simulink model "sampleModel1591"  (R2023a)
settings: Solver=VariableStepAuto  StartTime=0.0  StopTime=10.0  RelTol=1e-3
libraries: hdlsllib x7, simulink x2
settings Model: Creator=user1  LastModifiedBy=user1

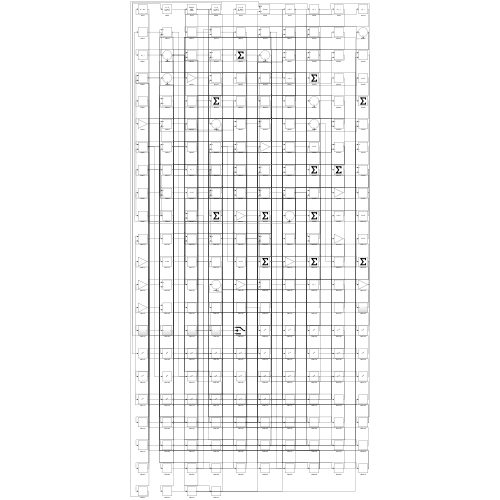
[thumbnail: Simulink's stored preview of the top-level diagram]
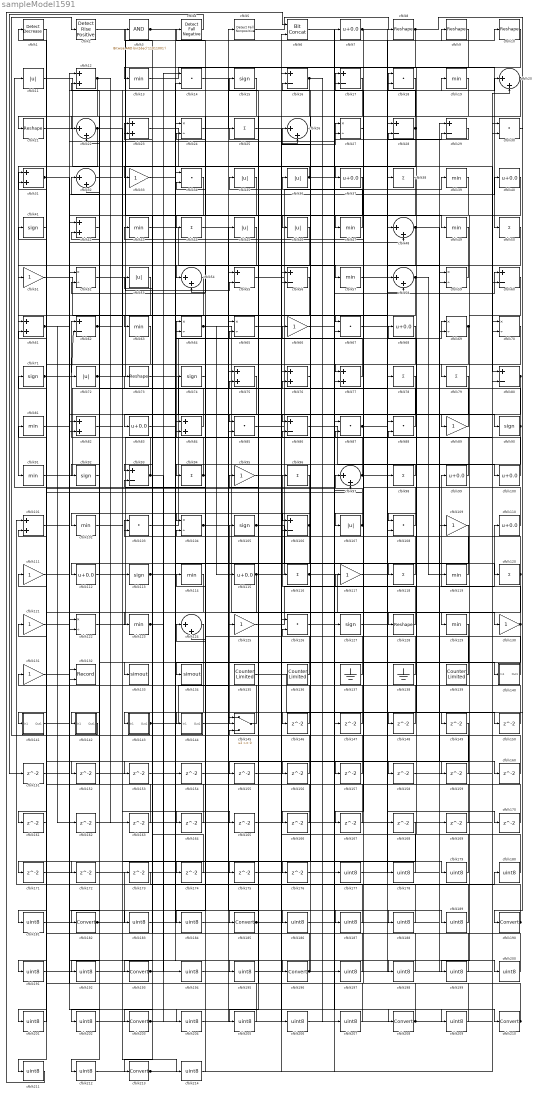
== system sampleModel1591 ==
  cfblk1 : simulink/Logic and Bit Operations/Detect Decrease  vinit=0.0  OutDataTypeStr=boolean
      settings: LibrarySourceBlock=|
      | hdlsllib/Logic and Bit
      | Operations/Detect
      | Decrease
  cfblk{8..10,21,73,128} (6 alike) : Reshape
  cfblk{7,37,40,68,83,99..100,110,112,115} (10 alike) : Bias  Bias=0.0  SaturateOnIntegerOverflow=off
  cfblk{12,23,31,42,61,75..77,82,84,101} (11 alike) : Sum
  cfblk{13,19,39,43,47,49,57,63,81,91,102,114,119,123,129} (15 alike) : MinMax
  cfblk{14,18,30,34,67,85,87..88,103,108,126} (11 alike) : DotProduct  OutDataTypeStr=Inherit: Inherit via internal rule
  cfblk{24,27,52,59,64..65,69..70,104,122} (10 alike) : Product  Inputs=*/  RndMeth=Zero  SaturateOnIntegerOverflow=on
  cfblk{15,41,71,74,90,92,105,113,127} (9 alike) : Signum
  cfblk{16..17,28..29,55..56,60,62,80,86,93,106} (12 alike) : Sum  Inputs=+-
  cfblk{11,35..36,45..46,53,72,107} (8 alike) : Abs  SaturateOnIntegerOverflow=off
  cfblk{33,51,66,89,95,109,111,117,121,125,130..131} (12 alike) : Gain
  cfblk{25,38,44,50,78..79,94,96,98,116,118,120} (12 alike) : Sum  Inputs=+
  cfblk{20,22,26,32,48,54,58,97,124} (9 alike) : Sum  Inputs=|++
  cfblk132 : Record  FileSettingsInternal="{\"entries\":[{\"content\":{\"excelSettings\":{\"content\":{},\"type\":\"Streamout.ExcelSettings\"}},\"type\":\"Streamout.FileSettingStorage\",\"uuid\":\"\"}],\"packageUris\":[\"http:\\/\\/schema.mathworks.com\\/mf0\\/streamout_blocks\\/R2020a\"],\"version\":\"1.0\"}"  Layout=[1 1]  SignalsInternal="{\"entries\":[{\"content\":{\"signals\":[{\"content\":{\"blockPath\":[],\"dimensions\":[1],\"domain\":\"\",\"lineColor\":\"#a2142f\",\"plots\":[1],\"port\":1,\"signalID\":2166,\"signalName\":\"XY Graph:1\"},\"type\":\"RecordBlkView.Signal\",\"uuid\":\"\"},{\"content\":{\"blockPath\":[],\"dimensions\":[1],\"domain\":\"\",\"lineColor\":\"#139fff\",\"plots\":[1],\"port\":2,\"signalID\":2169,\"signalName\":\"XY Graph:2\"},\"type\":\"RecordBlkView.Signal\",\"uuid\":\"\"}]},\"type\":\"RecordBlkView.InputSignals\",\"uuid\":\"\"}],\"packageUris\":[\"http:\\/\\/schema.mathworks.com\\/mf0\\/streamout_blocks\\/R2020a\"],\"version\":\"1.0\"}"  VisualizationBindings="{\"xyplotplugin\":{\"info\":[{\"series\":[{\"bindingParametersList\":[{\"parameter\":\"X-Axis\",\"signalID\":2166,\"signalName\":\"XY Graph:1\"},{\"parameter\":\"Y-Axis\",\"signalID\":2169,\"signalName\":\"XY Graph:2\"}],\"seriesID\":32629}],\"subplotID\":1}]}}"  CompatibilityTag=XY  st=-1
  cfblk133 : ToWorkspace  VariableName=simout  SaveFormat=Timeseries  SampleTime=-1
  cfblk134 : ToWorkspace  VariableName=simout  SaveFormat=Timeseries  SampleTime=-1
  cfblk135 : hdlsllib/Sources/Counter Limited  uplimit=7  tsamp=-1
  cfblk136 : hdlsllib/Sources/Counter Limited  uplimit=7  tsamp=-1
  cfblk137 : Ground
  cfblk138 : Ground
  cfblk139 : hdlsllib/Sources/Counter Limited  uplimit=7  tsamp=-1
  cfblk140 : Subsystem
      settings: LibrarySourceBlock=|
      | hdlsllib/Ports &
      | Subsystems/Subsystem
  cfblk141 : Subsystem
      settings: LibrarySourceBlock=|
      | hdlsllib/Ports &
      | Subsystems/Subsystem
  cfblk142 : Subsystem
      settings: LibrarySourceBlock=|
      | hdlsllib/Ports &
      | Subsystems/Subsystem
  cfblk143 : Subsystem
      settings: LibrarySourceBlock=|
      | hdlsllib/Ports &
      | Subsystems/Subsystem
  cfblk144 : Subsystem
      settings: LibrarySourceBlock=|
      | hdlsllib/Ports &
      | Subsystems/Subsystem
  cfblk145 : Switch  SaturateOnIntegerOverflow=off  InputSameDT=off
  cfblk{146..176} (31 alike) : Delay  SampleTime=1
  cfblk{177..181,183..184,186..189,191..192,194..195,197..202,204..207,209,211..212,214} (29 alike) : DataTypeConversion  OutDataTypeStr=uint8  SaturateOnIntegerOverflow=off  RndMeth=Floor
  cfblk{182,185,190,193,196,203,208,210,213} (9 alike) : DataTypeConversion  SaturateOnIntegerOverflow=off  RndMeth=Floor
  cfblk2 : hdlsllib/Logic and Bit Operations/Detect Rise Positive  vinit=0  OutDataTypeStr=boolean
  cfblk3 : simulink/Logic and Bit Operations/Bitwise Operator  logicop=AND  UseBitMask=on  BitMask=bin2dec('11011001')  BitMaskRealWorld=Stored Integer
      settings: LibrarySourceBlock=|
      | hdlsllib/Logic and Bit
      | Operations/Bitwise
      | Operator
  cfblk4 : hdlsllib/Logic and Bit Operations/Detect Fall Negative  vinit=0  OutDataTypeStr=boolean
  cfblk5 : hdlsllib/Logic and Bit Operations/Detect Fall Nonpositive  vinit=0  OutDataTypeStr=boolean
  cfblk6 : hdlsllib/Logic and Bit Operations/Bit Concat  numInputs=2
  wires:
  cfblk22/1 -> cfblk91/1, cfblk85/1, cfblk165/1, cfblk200/1
  cfblk100/1 -> cfblk62/1
  cfblk105/1 -> cfblk118/1, cfblk27/2
  cfblk115/1 -> cfblk39/1, cfblk123/1
  cfblk72/1 -> cfblk9/1, cfblk20/1
  cfblk13/1 -> cfblk50/1
  cfblk5/1 -> cfblk8/1
  cfblk137/1 -> cfblk11/1
  cfblk125/1 -> cfblk110/1
  cfblk73/1 -> cfblk90/1
  cfblk75/1 -> cfblk193/1
  cfblk108/1 -> cfblk43/1
  cfblk114/1 -> cfblk213/1
  cfblk42/1 -> cfblk112/1
  cfblk1/1 -> cfblk21/1
  cfblk122/1 -> cfblk97/1
  cfblk71/1 -> cfblk62/2, cfblk183/1
  cfblk64/1 -> cfblk130/1, cfblk115/1
  cfblk53/1 -> cfblk141/1(In1)
  cfblk116/1 -> cfblk129/1, cfblk60/1
  cfblk8/1 -> cfblk143/1(In1), cfblk13/1
  cfblk78/1 -> cfblk107/1
  cfblk107/1 -> cfblk31/1, cfblk71/1
  cfblk89/1 -> cfblk64/1
  cfblk113/1 -> cfblk69/1, cfblk195/1
  cfblk103/1 -> cfblk29/1
  cfblk92/1 -> cfblk142/1(In1)
  cfblk59/1 -> cfblk54/1
  cfblk99/1 -> cfblk74/1
  cfblk128/1 -> cfblk96/1
  cfblk16/1 -> cfblk44/1, cfblk205/1, cfblk207/1
  cfblk140/1(Out1) -> cfblk68/1
  cfblk145/1 -> cfblk81/1
  cfblk2/1 -> cfblk49/1
  cfblk90/1 -> cfblk16/2, cfblk148/1
  cfblk76/1 -> cfblk106/1
  cfblk12/1 -> cfblk61/1, cfblk163/1
  cfblk131/1 -> cfblk196/1
  cfblk69/1 -> cfblk77/1, cfblk122/2
  cfblk34/1 -> cfblk63/1
  cfblk48/1 -> cfblk133/1, cfblk132/2, cfblk160/1
  cfblk51/1 -> cfblk98/1
  cfblk83/1 -> cfblk84/1
  cfblk142/1(Out1) -> cfblk2/1
  cfblk47/1 -> cfblk15/1
  cfblk93/1 -> cfblk72/1, cfblk194/1
  cfblk14/1 -> cfblk89/1
  cfblk118/1 -> cfblk64/2
  cfblk21/1 -> cfblk80/1
  cfblk87/1 -> cfblk149/1, cfblk150/1
  cfblk38/1 -> cfblk46/1
  cfblk23/1 -> cfblk78/1
  cfblk10/1 -> cfblk128/1
  cfblk81/1 -> cfblk42/1
  cfblk20/1 -> cfblk166/1, cfblk167/1
  cfblk28/1 -> cfblk18/1, cfblk156/1
  cfblk84/1 -> cfblk32/2
  cfblk80/1 -> cfblk83/1, cfblk145/2
  cfblk117/1 -> cfblk48/1
  cfblk129/1 -> cfblk134/1
  cfblk55/1 -> cfblk57/1
  cfblk112/1 -> cfblk70/1
  cfblk104/1 -> cfblk24/2, cfblk186/1
  cfblk31/1 -> cfblk27/1, cfblk48/2
  cfblk43/1 -> cfblk127/1
  cfblk124/1 -> cfblk203/1
  cfblk91/1 -> cfblk76/2
  cfblk86/1 -> cfblk100/1
  cfblk24/1 -> cfblk5/1
  cfblk144/1(Out1) -> cfblk105/1
  cfblk74/1 -> cfblk4/1
  cfblk130/1 -> cfblk99/1, cfblk152/1
  cfblk85/1 -> cfblk28/1
  cfblk58/1 -> cfblk104/1, cfblk119/1, cfblk174/1
  cfblk60/1 -> cfblk79/1
  cfblk29/1 -> cfblk28/2
  cfblk3/1 -> cfblk140/1(In1), cfblk120/1
  cfblk57/1 -> cfblk58/2
  cfblk52/1 -> cfblk55/2
  cfblk123/1 -> cfblk103/1, cfblk154/1
  cfblk136/1 -> cfblk104/2
  cfblk11/1 -> cfblk97/2
  cfblk88/1 -> cfblk3/1
  cfblk120/1 -> cfblk53/1, cfblk181/1, cfblk184/1
  cfblk109/1 -> cfblk185/1
  cfblk94/1 -> cfblk23/1, cfblk144/1(In1)
  cfblk15/1 -> cfblk22/1
  cfblk62/1 -> cfblk113/1, cfblk18/2, cfblk175/1
  cfblk97/1 -> cfblk73/1, cfblk159/1
  cfblk61/1 -> cfblk40/1, cfblk41/1, cfblk85/2, cfblk162/1
  cfblk98/1 -> cfblk94/1
  cfblk110/1 -> cfblk84/2
  cfblk67/1 -> cfblk10/1
  cfblk141/1(Out1) -> cfblk17/1
  cfblk119/1 -> cfblk17/2
  cfblk121/1 -> cfblk82/1
  cfblk56/1 -> cfblk182/1
  cfblk7/1 -> cfblk37/1, cfblk59/2
  cfblk36/1 -> cfblk33/1, cfblk29/2
  cfblk26/1 -> cfblk86/1
  cfblk6/1 -> cfblk210/1
  cfblk9/1 -> cfblk47/1
  cfblk46/1 -> cfblk54/2
  cfblk35/1 -> cfblk82/2
  cfblk50/1 -> cfblk108/1
  cfblk54/1 -> cfblk93/1
  cfblk138/1 -> cfblk35/1
  cfblk111/1 -> cfblk208/1
  cfblk30/1 -> cfblk190/1
  cfblk32/1 -> cfblk19/1
  cfblk106/1 -> cfblk102/1, cfblk192/1
  cfblk143/1(Out1) -> cfblk125/1, cfblk179/1
  cfblk27/1 -> cfblk67/1
  cfblk49/1 -> cfblk51/1
  cfblk77/1 -> cfblk34/2
  cfblk139/1 -> cfblk52/2
  cfblk70/1 -> cfblk92/1
  cfblk19/1 -> cfblk146/1
  cfblk146/1 -> cfblk32/1
  cfblk66/1 -> cfblk147/1
  cfblk147/1 -> cfblk55/1
  cfblk148/1 -> cfblk34/1
  cfblk150/1 -> cfblk16/1
  cfblk4/1 -> cfblk151/1
  cfblk152/1 -> cfblk145/1
  cfblk39/1 -> cfblk153/1
  cfblk154/1 -> cfblk26/2
  cfblk18/1 -> cfblk155/1
  cfblk155/1 -> cfblk76/1
  cfblk156/1 -> cfblk31/2
  cfblk79/1 -> cfblk157/1
  cfblk157/1 -> cfblk106/2
  cfblk44/1 -> cfblk158/1
  cfblk158/1 -> cfblk80/2
  cfblk159/1 -> cfblk12/2
  cfblk160/1 -> cfblk86/2
  cfblk41/1 -> cfblk161/1
  cfblk161/1 -> cfblk61/2
  cfblk162/1 -> cfblk77/2
  cfblk163/1 -> cfblk22/2
  cfblk102/1 -> cfblk164/1
  cfblk164/1 -> cfblk24/1
  cfblk165/1 -> cfblk70/2
  cfblk166/1 -> cfblk42/2
  cfblk167/1 -> cfblk93/2
  cfblk169/1 -> cfblk145/3
  cfblk127/1 -> cfblk170/1
  cfblk170/1 -> cfblk1/1
  cfblk68/1 -> cfblk171/1
  cfblk171/1 -> cfblk69/2
  cfblk17/1 -> cfblk172/1
  cfblk172/1 -> cfblk58/1
  cfblk174/1 -> cfblk23/2
  cfblk175/1 -> cfblk67/2
  cfblk37/1 -> cfblk176/1
  cfblk176/1 -> cfblk7/1
  cfblk126/1 -> cfblk177/1
  cfblk177/1 -> cfblk59/1
  cfblk135/1 -> cfblk178/1
  cfblk178/1 -> cfblk126/1
  cfblk179/1 -> cfblk126/2
  cfblk173/1 -> cfblk180/1
  cfblk180/1 -> cfblk88/2
  cfblk181/1 -> cfblk173/1
  cfblk182/1 -> cfblk108/2, cfblk14/2
  cfblk183/1 -> cfblk56/1
  cfblk184/1 -> cfblk56/2
  cfblk185/1 -> cfblk116/1, cfblk88/1
  cfblk186/1 -> cfblk109/1
  cfblk101/1 -> cfblk187/1
  cfblk187/1 -> cfblk95/1
  cfblk153/1 -> cfblk188/1
  cfblk188/1 -> cfblk101/1
  cfblk33/1 -> cfblk189/1
  cfblk189/1 -> cfblk101/2
  cfblk190/1 -> cfblk12/1, cfblk66/1
  cfblk149/1 -> cfblk191/1
  cfblk191/1 -> cfblk30/1
  cfblk192/1 -> cfblk30/2
  cfblk193/1 -> cfblk169/1, cfblk168/1
  cfblk194/1 -> cfblk75/1
  cfblk195/1 -> cfblk75/2
  cfblk196/1 -> cfblk103/2, cfblk38/1, cfblk26/1
  cfblk197/1 -> cfblk131/1
  cfblk65/1 -> cfblk198/1
  cfblk198/1 -> cfblk36/1
  cfblk40/1 -> cfblk199/1
  cfblk199/1 -> cfblk65/1
  cfblk200/1 -> cfblk65/2
  cfblk45/1 -> cfblk201/1
  cfblk201/1 -> cfblk121/1
  cfblk96/1 -> cfblk202/1
  cfblk202/1 -> cfblk45/1
  cfblk203/1 -> cfblk60/2, cfblk14/1
  cfblk151/1 -> cfblk204/1
  cfblk204/1 -> cfblk124/1
  cfblk205/1 -> cfblk124/2
  cfblk25/1 -> cfblk206/1
  cfblk206/1 -> cfblk87/1
  cfblk207/1 -> cfblk25/1
  cfblk208/1 -> cfblk87/2, cfblk117/1, cfblk122/1
  cfblk95/1 -> cfblk209/1
  cfblk209/1 -> cfblk111/1
  cfblk210/1 -> cfblk132/1, cfblk52/1
  cfblk168/1 -> cfblk211/1
  cfblk211/1 -> cfblk6/1
  cfblk63/1 -> cfblk212/1
  cfblk212/1 -> cfblk6/2
  cfblk213/1 -> cfblk197/1, cfblk20/2
  cfblk82/1 -> cfblk214/1
  cfblk214/1 -> cfblk114/1

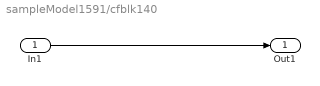
== system sampleModel1591/cfblk140 ==
  In1 : Inport
  Out1 : Outport
  wires:
  In1/1 -> Out1/1

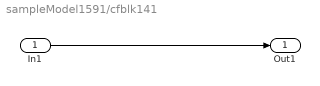
== system sampleModel1591/cfblk141 ==
  In1 : Inport
  Out1 : Outport
  wires:
  In1/1 -> Out1/1

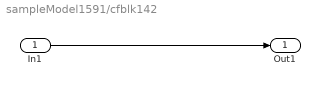
== system sampleModel1591/cfblk142 ==
  In1 : Inport
  Out1 : Outport
  wires:
  In1/1 -> Out1/1

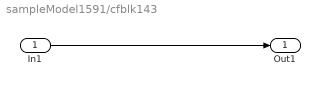
== system sampleModel1591/cfblk143 ==
  In1 : Inport
  Out1 : Outport
  wires:
  In1/1 -> Out1/1

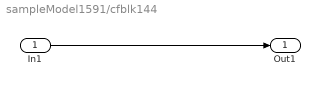
== system sampleModel1591/cfblk144 ==
  In1 : Inport
  Out1 : Outport
  wires:
  In1/1 -> Out1/1
